simulink model "bepf_drivre"  (R2016b)
settings: Solver=VariableStepAuto  StartTime=0.0  StopTime=50  RelTol=1e-3
libraries: vrlib x2
settings Model: Creator=gagato  LastModifiedBy=gagato

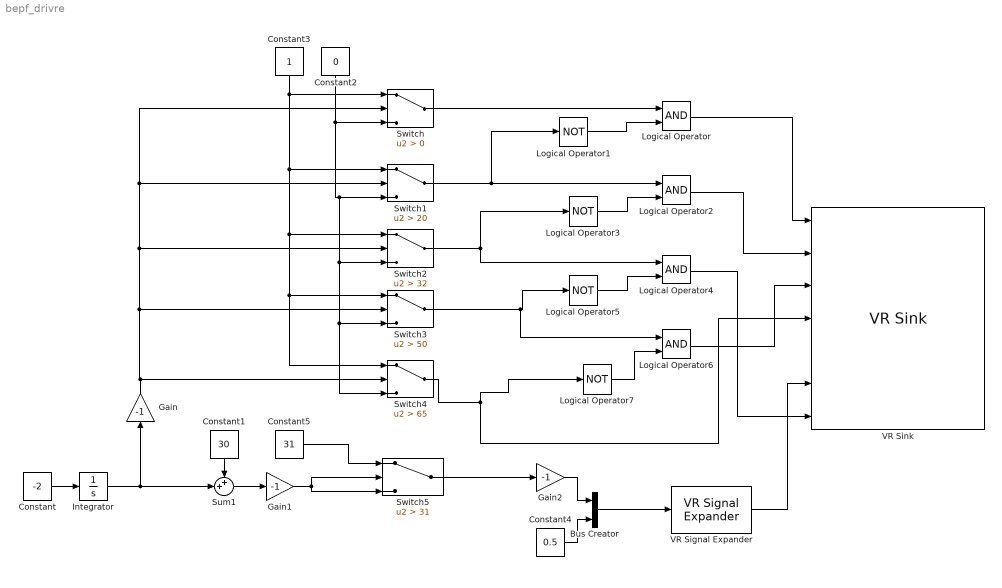
== system bepf_drivre ==
  Bus Creator : BusCreator  Inputs=2
  Constant : Constant  Value=-2
  Constant1 : Constant  Value=30
  Constant2 : Constant  Value=0
  Constant3 : Constant
  Constant4 : Constant  Value=0.5
  Constant5 : Constant  Value=31
  Gain : Gain  Gain=-1
  Gain1 : Gain  Gain=-1
  Gain2 : Gain  Gain=-1
  Integrator : Integrator
  Logical Operator{,2,4,6} (4 alike) : Logic  AllPortsSameDT=off  OutDataTypeStr=boolean
  Logical Operator{1,3,5,7} (4 alike) : Logic  Operator=NOT  AllPortsSameDT=off  OutDataTypeStr=boolean
  Sum1 : Sum  Inputs=++|
  Switch : Switch  Criteria=u2 > Threshold
  Switch1 : Switch  Criteria=u2 > Threshold  Threshold=20
  Switch2 : Switch  Criteria=u2 > Threshold  Threshold=32
  Switch3 : Switch  Criteria=u2 > Threshold  Threshold=50
  Switch4 : Switch  Criteria=u2 > Threshold  Threshold=65
  Switch5 : Switch  Criteria=u2 > Threshold  Threshold=31
  VR Signal Expander : vrlib/VR Signal Expander  outwidth=3  outidx=[1 3]
  VR Sink : vrlib/VR Sink  InstantiateOnLoad=on  SampleTime=0.1  ViewEnable=on  RemoteChange=off  RemoteView=off  FieldsWritten=Pierwszy.set_bind.1.1.1.logical#Drugi.set_bind.1.1.1.logical#Czwarty.set_bind.1.1.1.logical#Piaty.set_bind.1.1.1.logical#Bepf.rotation.4.1.1.double#Bepf.translation.3.1.1.double#Trzy.set_bind.1.1.1.logical  WorldFileName=bepf_drivre.wrl  AutoView=off  VideoDimensions=[]  AllowVariableSize=off
  wires:
  Constant/1 -> Integrator/1
  Integrator/1 -> Sum1/2, Gain/1
  VR Signal Expander/1 -> VR Sink/6
  Constant3/1 -> Switch1/1, Switch2/1, Switch3/1, Switch4/1, Switch/1
  Constant2/1 -> Switch/3, Switch1/3, Switch3/3, Switch4/3, Switch2/3
  Switch1/1 -> Logical Operator2/1, Logical Operator1/1
  Switch2/1 -> Logical Operator3/1, Logical Operator4/1
  Switch4/1 -> Logical Operator7/1, VR Sink/4
  Constant1/1 -> Sum1/1
  Sum1/1 -> Gain1/1
  Gain/1 -> Switch3/2, Switch2/2, Switch1/2, Switch/2, Switch4/2
  Logical Operator1/1 -> Logical Operator/2
  Logical Operator/1 -> VR Sink/1
  Switch/1 -> Logical Operator/1
  Logical Operator2/1 -> VR Sink/2
  Logical Operator3/1 -> Logical Operator2/2
  Logical Operator5/1 -> Logical Operator4/2
  Switch3/1 -> Logical Operator6/1, Logical Operator5/1
  Logical Operator4/1 -> VR Sink/7
  Logical Operator6/1 -> VR Sink/3
  Logical Operator7/1 -> Logical Operator6/2
  Bus Creator/1 -> VR Signal Expander/1
  Constant4/1 -> Bus Creator/2
  Constant5/1 -> Switch5/1
  Switch5/1 -> Gain2/1
  Gain1/1 -> Switch5/3, Switch5/2
  Gain2/1 -> Bus Creator/1
